simulink library "temp"  (Simulink 5.0)
undefined symbols (not defined in the file or in its folder): A, A1, B, B1, C, C1, D, D1, F, H, matrix, v1_vec, v2_vec, v3_vec, v_vec
libraries: aerolibschedule x46, simulink3 x46, simulink x18
(part 1 of 2)
settings Model: Creator=sgage  LastModifiedBy=sgage  ExtModeAutoUpdateStatusClock=off

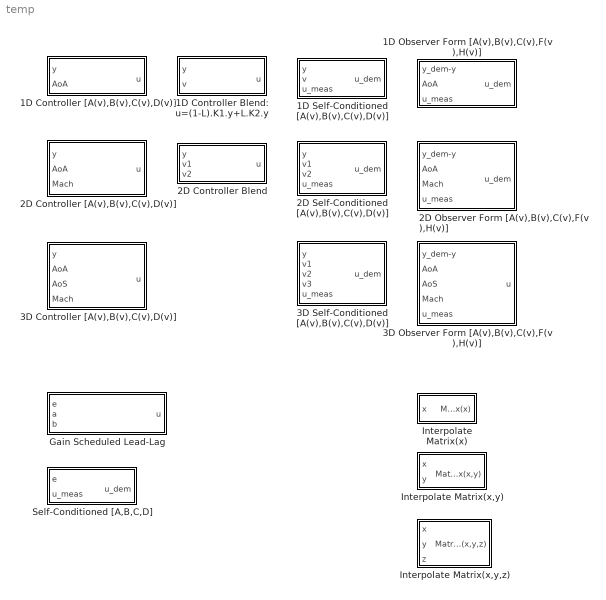
== system temp ==
  1D Controller [A(v),B(v),C(v),D(v)] : Subsystem  mask(StateSpaceABCD-1D){A=A1, B=B1, C=C1, D=D1, AoA_vec=v_vec, x_initial=0}
      mask prompts: A "A-matrix(v):"; B "B-matrix(v):"; C "C-matrix(v):"; D "D-matrix(v):"; AoA_vec "Scheduling variable breakpoints:"; x_initial "Initial state, x_initial:"
      mask help: Implement a state-space controller [A,B,C,D] where A, B, C, and D depend on one scheduling parameter, v.
      mask Help: web(asbhelp('1dcontrolleravbvcvdv'));
      mask Display:
      | port_label('input',1,'y');
      | port_label('input',2,'v');
      | port_label('output',1,'u');
  1D Controller Blend: u=(1-L).K1.y+L.K2.y : Subsystem  mask(Blend-1D){A=A1, B=B1, C=C1, D=D1, breakpoints_v=[1 1.5 2], x_initial=0, vec_w=[-5 -2]}
      mask prompts: A "A-matrix(v):"; B "B-matrix(v):"; C "C-matrix(v):"; D "D-matrix(v):"; breakpoints_v "Scheduling variable breakpoints:"; x_initial "Initial state, x_initial:"; vec_w "Poles of A(v)-H(v)*C(v) = [w1 ... wn]:"
      mask help: Blend between outputs of a 1-D vector of state-space controllers. All controllers must have the same state dimension.
      mask init:
      | for i=1:length(breakpoints_v);
      |     L1 = place(squeeze(A(:,:,i))',squeeze(C(:,:,i))',vec_w);
      |     H(:,:,i)=L1';
      | end
      mask Help: web(asbhelp('1dcontrollerblendu1l.k1.yl.k2.y'));
  1D Observer Form [A(v),B(v),C(v),F(v),H(v)] : Subsystem  mask(StateSpaceABCFH-1D){A=A, B=B, C=C, F=F, H=H, AoA_vec=v_vec, x_initial=0}
      mask prompts: A "A-matrix(v):"; B "B-matrix(v):"; C "C-matrix(v):"; F "F-matrix(v):"; H "H-matrix(v):"; AoA_vec "Scheduling variable breakpoints:"; x_initial "Initial state, x_initial:"
      mask help: Implement a state-space controller [A,B,C,F,H] in observer form where A, B, C, F, and H depend on one scheduling parameter.
      mask Help: web(asbhelp('1dobserverformavbvcvfvhv'));
      mask Display:
      | port_label('input',1,'y-y_dem');
      | port_label('input',2,'v');
      | port_label('input',3,'u_meas');
      | port_label('output',1,'u_dem')
  1D Self-Conditioned [A(v),B(v),C(v),D(v)] : Subsystem  mask(StateSpaceSelfCond-1D){A=A, B=B, C=C, D=D, breakpoints_v=v_vec, x_initial=0, vec_w=[-5 -2]}
      mask prompts: A "A-matrix(v):"; B "B-matrix(v):"; C "C-matrix(v):"; D "D-matrix(v):"; breakpoints_v "Scheduling variable breakpoints:"; x_initial "Initial state, x_initial:"; vec_w "Poles of A(v)-H(v)*C(v) = [w1 ... wn]:"
      mask help: Implement a state-space controller [A(v),B(v),C(v),D(v)] in a self-conditioned form. If u_meas = u_dem, then the implemented controller is [A,B,C,D]. If u_meas is limited, e.g., rate limiting, then the poles of the controller become those defined in the mask dialog box. Uses call to Control Systems Toolbox function place.m when initializing. A, B, C, and D should be 3-D matrices, the last dimension corresponding to the scheduling parameter, and the first two corresponding to the matrix for a given set of scheduling parameter values.
      mask init:
      | for i=1:length(breakpoints_v);
      |     L1 = place(squeeze(A(:,:,i))',squeeze(C(:,:,i))',vec_w);
      |     H(:,:,i)=L1';
      | end
      mask Help: web(asbhelp('1dselfconditionedavbvcvdv'));
  2D Controller [A(v),B(v),C(v),D(v)] : Subsystem  mask(StateSpaceABCD-2D){A=A, B=B, C=C, D=D, AoA_vec=v1_vec, Mach_vec=v2_vec, x_initial=0}
      mask prompts: A "A-matrix(v1,v2):"; B "B-matrix(v1,v2):"; C "C-matrix(v1,v2):"; D "D-matrix(v1,v2):"; AoA_vec "First scheduling variable (v1) breakpoints:"; Mach_vec "Second scheduling variable (v2) breakpoints:"; x_initial "Initial state, x_initial:"
      mask help: Implement a state-space controller [A,B,C,D] where A, B, C, and D depend on two scheduling parameters, v1 and v2.
      mask Help: web(asbhelp('2dcontrolleravbvcvdv'));
      mask Display:
      | port_label('input',1,'y');
      | port_label('input',2,'v1');
      | port_label('input',3,'v2');
      | port_label('output',1,'u');
  2D Controller Blend : Subsystem  mask(Blend-2D){A=A, B=B, C=C, D=D, breakpoints_v1=v1_vec, breakpoints_v2=v2_vec, x_initial=0, vec_w=[-5 -2]}
      mask prompts: A "A-matrix(v1,v2):"; B "B-matrix(v1,v2):"; C "C-matrix(v1,v2):"; D "D-matrix(v1,v2):"; breakpoints_v1 "First scheduling variable (v1) breakpoints:"; breakpoints_v2 "Second scheduling variable (v2) breakpoints:"; x_initial "Initial state, x_initial:"; vec_w "Poles of A(v)-H(v)*C(v) = [w1 ... wn]:"
      mask help: Blend between outputs of a 2-D vector of state-space controllers. All controllers must have the same state dimension.
      mask init:
      | for i=1:length(breakpoints_v1);
      |   for j=1:length(breakpoints_v2);
      |     L1 = place(squeeze(A(:,:,i,j))',squeeze(C(:,:,i,j))',vec_w);
      |     H(:,:,i,j)=L1';
      |   end
      | end
      mask Help: web(asbhelp('2dcontrollerblend'));
  2D Observer Form [A(v),B(v),C(v),F(v),H(v)] : Subsystem  mask(StateSpaceABCFH-2D){A=A, B=B, C=C, F=F, H=H, AoA_vec=v1_vec, Mach_vec=v2_vec, x_initial=0}
      mask prompts: A "A-matrix(v1,v2):"; B "B-matrix(v1,v2):"; C "C-matrix(v1,v2):"; F "F-matrix(v1,v2):"; H "H-matrix(v1,v2):"; AoA_vec "First scheduling variable (v1) breakpoints:"; Mach_vec "Second scheduling variable (v2) breakpoints:"; x_initial "Initial state, x_initial:"
      mask help: Implement a state-space controller [A,B,C,F,H] in observer form where A, B, C, F, and H depend on two scheduling parameters.
      mask Help: web(asbhelp('2dobserverformavbvcvfvhv'));
      mask Display:
      | port_label('input',1,'y-y_dem');
      | port_label('input',2,'v1');
      | port_label('input',3,'v2');
      | port_label('input',4,'u_meas');
      | port_label('output',1,'u_dem')
  2D Self-Conditioned [A(v),B(v),C(v),D(v)] : Subsystem  mask(StateSpaceSelfCond-2D){A=A, B=B, C=C, D=D, breakpoints_v1=v1_vec, breakpoints_v2=v2_vec, x_initial=0, vec_w=[-5 -2]}
      mask prompts: A "A-matrix(v1,v2):"; B "B-matrix(v1,v2):"; C "C-matrix(v1,v2):"; D "D-matrix(v1,v2):"; breakpoints_v1 "First scheduling variable (v1) breakpoints:"; breakpoints_v2 "Second scheduling variable (v2) breakpoints:"; x_initial "Initial state, x_initial:"; vec_w "Poles of A(v)-H(v)*C(v) = [w1 ... wn]:"
      mask help: Implement a state-space controller [A(v1,v2),B(v1,v2),C(v1,v2),D(v1,v2)] in a self-conditioned form. If u_meas = u_dem, then the implemented controller is [A,B,C,D]. If u_meas is limited, e.g., rate limiting, then the poles of the controller become those defined in the mask dialog box. Uses call to Control Systems Toolbox function place.m when initializing. A, B, C, and D should be 4-D matrices, the last two dimensions corresponding to the scheduling parameters, and the first two corresponding to the matrix for a given set of scheduling parameter values.
      mask init:
      | for i=1:length(breakpoints_v1);
      |   for j=1:length(breakpoints_v2);
      |     L1 = place(squeeze(A(:,:,i,j))',squeeze(C(:,:,i,j))',vec_w);
      |     H(:,:,i,j)=L1';
      |   end
      | end
      mask Help: web(asbhelp('2dselfconditionedavbvcvdv'));
  3D Controller [A(v),B(v),C(v),D(v)] : Subsystem  mask(StateSpaceABCD-3D){A=A, B=B, C=C, D=D, AoA_vec=v1_vec, AoS_vec=v2_vec, Mach_vec=v3_vec, x_initial=0}
      mask prompts: A "A-matrix(v1,v2,v3):"; B "B-matrix(v1,v2,v3):"; C "C-matrix(v1,v2,v3):"; D "D-matrix(v1,v2,v3):"; AoA_vec "First scheduling variable (v1) breakpoints:"; AoS_vec "Second scheduling variable (v2) breakpoints:"; Mach_vec "Third scheduling variable (v3) breakpoints:"; x_initial "Initial state, x_initial:"
      mask help: Implement a state-space controller [A,B,C,D] where A, B, C, and D depend on three scheduling parameters, v1, v2, and v3.
      mask Help: web(asbhelp('3dcontrolleravbvcvdv'));
      mask Display:
      | port_label('input',1,'y');
      | port_label('input',2,'v1');
      | port_label('input',3,'v2');
      | port_label('input',4,'v3');
      | port_label('output',1,'u');
  3D Observer Form [A(v),B(v),C(v),F(v),H(v)] : Subsystem  mask(StateSpaceABCFH-3D){A=A, B=B, C=C, F=F, H=H, AoA_vec=v1_vec, AoS_vec=v2_vec, Mach_vec=v3_vec, x_initial=0}
      mask prompts: A "A-matrix(v1,v2,v3):"; B "B-matrix(v1,v2,v3):"; C "C-matrix(v1,v2,v3):"; F "F-matrix(v1,v2,v3):"; H "H-matrix(v1,v2,v3):"; AoA_vec "First scheduling variable (v1) breakpoints:"; AoS_vec "Second scheduling variable (v2) breakpoints:"; Mach_vec "Third scheduling variable (v3) breakpoints:"; x_initial "Initial state, x_initial:"
      mask help: Implement a state-space controller [A,B,C,F,H] in observer form where A, B, C, F, and H depend on three scheduling parameters.
      mask Help: web(asbhelp('3dobserverformavbvcvfvhv'));
      mask Display:
      | port_label('input',1,'y-y_dem');
      | port_label('input',2,'v1');
      | port_label('input',3,'v2');
      | port_label('input',4,'v3');
      | port_label('input',5,'u_meas');
      | port_label('output',1,'u_dem')
  3D Self-Conditioned [A(v),B(v),C(v),D(v)] : Subsystem  mask(StateSpaceSelfCond-3D){A=A, B=B, C=C, D=D, breakpoints_v1=v1_vec, breakpoints_v2=v2_vec, breakpoints_v3=v3_vec, x_initial=0, vec_w=[-5 -2]}
      mask prompts: A "A-matrix(v1,v2,v3):"; B "B-matrix(v1,v2,v3):"; C "C-matrix(v1,v2,v3):"; D "D-matrix(v1,v2,v3):"; breakpoints_v1 "First scheduling variable (v1) breakpoints:"; breakpoints_v2 "Second scheduling variable (v2) breakpoints:"; breakpoints_v3 "Third scheduling variable (v3) breakpoints:"; x_initial "Initial state, x_initial:"; vec_w "Poles of A(v)-H(v)*C(v) = [w1 ... wn]:"
      mask help: Implement a state-space controller [A(v1,v2,v3),B(v1,v2,v3),C(v1,v2,v3),D(v1,v2,v3)] in a self-conditioned form. If u_meas = u_dem, then the implemented controller is [A,B,C,D]. If u_meas is limited, e.g., rate limiting, then the poles of the controller become those defined in the mask dialog box. Uses call to Control Systems Toolbox function place.m when initializing. A, B, C, and D should be 5-D matrices, the last three dimensions corresponding to the scheduling parameters, and the first two corresponding to the matrix for a given set of scheduling parameter values.
      mask init:
      | for i=1:length(breakpoints_v1);
      |   for j=1:length(breakpoints_v2);
      |     for k=1:length(breakpoints_v3);
      |       L1 = place(squeeze(A(:,:,i,j,k))',squeeze(C(:,:,i,j,k))',vec_w);
      |       H(:,:,i,j,k)=L1';
      |     end
      |   end
      | end
      mask Help: web(asbhelp('3dselfconditionedavbvcvdv'));
  Gain Scheduled Lead-Lag : Subsystem  mask(Gain Scheduled Lead-Lag){x_initial=0}
      mask prompts: x_initial "Initial state, x_initial:"
      mask help: Implement gain-scheduled first-order lead-lag of the form [1+a.s]/[1+b.s]. Initial output is given by (x_initial+a.e)/b where x_initial is the initial state defined in the mask dialog box. Note that b should never be allowed to be zero.
      mask Help: web(asbhelp);
      mask Display:
      | port_label('input',1,'e');
      | port_label('input',2,'a');
      | port_label('input',3,'b');
      | port_label('output',1,'u');
      | disp('(1+a.s)/(1+b.s)')
  Interpolate Matrix(x) : Subsystem  mask(MatrixSchedule-1D){matrix=matrix}
      mask prompts: matrix "Matrix to interpolate:"
      mask help: Return an interpolated matrix for given input x. Input x must be from the Simulink PreLook-up Index Search block.
      mask Help: web(asbhelp('interpolatematrixx'));
  Interpolate Matrix(x,y) : Subsystem  mask(MatrixSchedule-2D){matrix=matrix}
      mask prompts: matrix "Matrix to interpolate:"
      mask help: Return an interpolated matrix for given inputs x and y. Inputs x and y must be from Simulink PreLook-up Index Search block.
      mask Help: web(asbhelp('interpolatematrixxy'));
  Interpolate Matrix(x,y,z) : Subsystem  mask(MatrixSchedule-3D){matrix=matrix}
      mask prompts: matrix "Matrix to interpolate:"
      mask help: Return an interpolated matrix for given inputs x, y, and z. Inputs x, y, z must be from Simulink PreLook-up Index Search block.
      mask Help: web(asbhelp('interpolatematrixxyz'));
  Self-Conditioned [A,B,C,D] : Subsystem  mask(Self-Conditioned){Ak=[-1 -0.2;0 -3], Bk=[1;1], Ck=[1 0], Dk=0.02, x_initial=0, vec_w=[-5 -2]}
      mask prompts: Ak "A-matrix:"; Bk "B-matrix:"; Ck "C-matrix:"; Dk "D-matrix:"; x_initial "Initial state, x_initial:"; vec_w "Poles of A-H*C = [w1 ... wn]:"
      mask help: Implement a state-space controller [A,B,C,D] in a self-conditioned form. If u_meas = u_dem, then the implemented controller is [A,B,C,D]. If u_meas is limited, e.g., rate limiting, then the poles of the controller become those defined in the mask dialog box. Uses call to Control Systems Toolbox function place.m when initializing.
      mask init:
      | L1 = place(Ak',Ck',vec_w);
      | H=L1';
      mask Help: web(asbhelp('selfconditionedabcd'))

== system temp/1D Controller [A(v),B(v),C(v),D(v)] ==
  y : Inport
  AoA : Inport  Port=2  PortDimensions=1
  "[A,B,C,D]" : Subsystem
  alpha (degs) : simulink3/Functions & Tables/PreLook-Up Index Search  bpData=AoA_vec  searchMode=Binary Search  cacheBpFlag=on  outputFlag=off  extrapMode=Clip to Range  rangeErrorMode=None
  u : Outport
  wires:
  y/1 -> "[A,B,C,D]"/1(y)
  AoA/1 -> alpha (degs)/1
  alpha (degs)/1 -> "[A,B,C,D]"/2(AoA)
  "[A,B,C,D]"/1(u) -> u/1

== system temp/1D Controller Blend: u=(1-L).K1.y+L.K2.y ==
  y : Inport
  v : Inport  Port=2  PortDimensions=1
  Breakpoints : simulink/Look-Up Tables/PreLook-Up Index Search  bpData=breakpoints_v  searchMode=Binary Search  cacheBpFlag=on  outputFlag=off  extrapMode=Clip to Range  rangeErrorMode=None
  Controller indices : Subsystem  AncestorBlock=|
      | aerolibschedule/1D Controller Blend:
      | u=(1-L).K1.y+L.K2.y/Controller indices
  Demux : Demux  Outputs=2
  K1 : Subsystem
  K2 : Subsystem
  K3 : Subsystem
  Sum1 : Sum  Inputs=+++  SaturateOnIntegerOverflow=on  InputSameDT=on
  lambda1 : Product  SaturateOnIntegerOverflow=on  InputSameDT=on
  lambda2 : Product  SaturateOnIntegerOverflow=on  InputSameDT=on
  lambda3 : Product  SaturateOnIntegerOverflow=on  InputSameDT=on
  u : Outport
  wires:
  Controller indices/6(lambda_K3) -> lambda3/2
  Controller indices/4(lambda_K2) -> lambda2/2
  Controller indices/2(lambda_K1) -> lambda1/2
  Sum1/1 -> K1/3(u_measured), K3/3(u_measured), K2/3(u_measured), u/1
  lambda3/1 -> Sum1/3
  lambda1/1 -> Sum1/1
  lambda2/1 -> Sum1/2
  K3/1(u_demand) -> lambda3/1
  K2/1(u_demand) -> lambda2/1
  K1/1(u_demand) -> lambda1/1
  Controller indices/5(idx_K3) -> K3/2(index)
  Controller indices/3(idx_K2) -> K2/2(index)
  Controller indices/1(idx_K1) -> K1/2(index)
  Demux/2 -> Controller indices/2(lambda)
  Demux/1 -> Controller indices/1(index)
  Breakpoints/1 -> Demux/1
  v/1 -> Breakpoints/1
  y/1 -> K1/1(e = refs - y), K3/1(e = refs - y), K2/1(e = refs - y)

== system temp/1D Observer Form [A(v),B(v),C(v),F(v),H(v)] ==
  y_dem-y : Inport
  AoA : Inport  Port=2  PortDimensions=1
  u_meas : Inport  Port=3
  Reshape : simulink3/Signals & Systems/Reshape  OutputDimensionality=1-D array  OutputDimensions=[1,1]
  Reshape1 : simulink3/Signals & Systems/Reshape  OutputDimensionality=Column vector  OutputDimensions=[1,1]
  Reshape2 : simulink3/Signals & Systems/Reshape  OutputDimensionality=Column vector  OutputDimensions=[1,1]
  "[A,B,C,F,H]" : Subsystem
  alpha (degs) : simulink3/Functions & Tables/PreLook-Up Index Search  bpData=AoA_vec  searchMode=Binary Search  cacheBpFlag=on  outputFlag=off  extrapMode=Clip to Range  rangeErrorMode=None
  u_dem : Outport
  wires:
  "[A,B,C,F,H]"/1(u_dem) -> Reshape/1
  AoA/1 -> alpha (degs)/1
  y_dem-y/1 -> Reshape2/1
  alpha (degs)/1 -> "[A,B,C,F,H]"/2(AoA)
  u_meas/1 -> Reshape1/1
  Reshape/1 -> u_dem/1
  Reshape1/1 -> "[A,B,C,F,H]"/3(u_meas)
  Reshape2/1 -> "[A,B,C,F,H]"/1(y-y_dem)

== system temp/1D Self-Conditioned [A(v),B(v),C(v),D(v)] ==
  y : Inport
  v : Inport  Port=2  PortDimensions=1
  u_meas : Inport  Port=3
  Breakpoints : simulink3/Functions & Tables/PreLook-Up Index Search  bpData=breakpoints_v  searchMode=Binary Search  cacheBpFlag=on  outputFlag=off  extrapMode=Clip to Range  rangeErrorMode=None
  Controller : Subsystem
  u_dem : Outport
  wires:
  v/1 -> Breakpoints/1
  y/1 -> Controller/1(y)
  Controller/1(u_demand) -> u_dem/1
  Breakpoints/1 -> Controller/2(idx_v,lam_v)
  u_meas/1 -> Controller/3(u_measured)

== system temp/2D Controller [A(v),B(v),C(v),D(v)] ==
  y : Inport
  AoA : Inport  Port=2  PortDimensions=1
  Mach : Inport  Port=3  PortDimensions=1
  Mach No. : simulink3/Functions & Tables/PreLook-Up Index Search  bpData=Mach_vec  searchMode=Binary Search  cacheBpFlag=on  outputFlag=off  extrapMode=Clip to Range  rangeErrorMode=None
  "[A,B,C,D]" : Subsystem
  alpha (degs) : simulink3/Functions & Tables/PreLook-Up Index Search  bpData=AoA_vec  searchMode=Binary Search  cacheBpFlag=on  outputFlag=off  extrapMode=Clip to Range  rangeErrorMode=None
  u : Outport
  wires:
  y/1 -> "[A,B,C,D]"/1(y)
  Mach/1 -> Mach No./1
  AoA/1 -> alpha (degs)/1
  Mach No./1 -> "[A,B,C,D]"/3(Mach)
  alpha (degs)/1 -> "[A,B,C,D]"/2(AoA)
  "[A,B,C,D]"/1(u) -> u/1

== system temp/2D Controller Blend ==
  y : Inport
  v1 : Inport  Port=2  PortDimensions=1
  v2 : Inport  Port=3  PortDimensions=1
  Breakpoints v1 : simulink/Look-Up Tables/PreLook-Up Index Search  bpData=breakpoints_v1  searchMode=Binary Search  cacheBpFlag=on  outputFlag=off  extrapMode=Clip to Range  rangeErrorMode=None
  Controller indices1 : Subsystem
  Demux : Demux  Outputs=2
  K1 : Subsystem
  K2 : aerolibschedule/2D Controller Blend/K1  SimViewingDevice=off  DataTypeOverride=UseLocalSettings  MinMaxOverflowLogging=UseLocalSettings
      settings: Permissions=ReadWrite  RTWFcnNameOpts=Auto  RTWFileNameOpts=Auto
  K3 : aerolibschedule/2D Controller Blend/K1  SimViewingDevice=off  DataTypeOverride=UseLocalSettings  MinMaxOverflowLogging=UseLocalSettings
      settings: Permissions=ReadWrite  RTWFcnNameOpts=Auto  RTWFileNameOpts=Auto
  Sum1 : Sum  Inputs=+++  SaturateOnIntegerOverflow=on  InputSameDT=on
  lambda1 : Product  SaturateOnIntegerOverflow=on  InputSameDT=on
  lambda2 : Product  SaturateOnIntegerOverflow=on  InputSameDT=on
  lambda3 : Product  SaturateOnIntegerOverflow=on  InputSameDT=on
  u : Outport
  wires:
  v2/1 -> K2/4, K3/4, K1/4(v2)
  Controller indices1/6(lambda_K3) -> lambda3/2
  Controller indices1/4(lambda_K2) -> lambda2/2
  Controller indices1/2(lambda_K1) -> lambda1/2
  Sum1/1 -> K2/3, K3/3, K1/3(u_measured), u/1
  lambda3/1 -> Sum1/3
  lambda1/1 -> Sum1/1
  lambda2/1 -> Sum1/2
  K3/1 -> lambda3/1
  K2/1 -> lambda2/1
  K1/1(u_demand) -> lambda1/1
  Controller indices1/5(idx_K3) -> K3/2
  Controller indices1/3(idx_K2) -> K2/2
  Controller indices1/1(idx_K1) -> K1/2(index_v1)
  Demux/2 -> Controller indices1/2(lambda)
  Demux/1 -> Controller indices1/1(index)
  Breakpoints v1/1 -> Demux/1
  v1/1 -> Breakpoints v1/1
  y/1 -> K2/1, K3/1, K1/1(e = refs - y)

== system temp/2D Observer Form [A(v),B(v),C(v),F(v),H(v)] ==
  y_dem-y : Inport
  AoA : Inport  Port=2  PortDimensions=1
  Mach : Inport  Port=3  PortDimensions=1
  u_meas : Inport  Port=4
  Mach No. : simulink3/Functions & Tables/PreLook-Up Index Search  bpData=Mach_vec  searchMode=Binary Search  cacheBpFlag=on  outputFlag=off  extrapMode=Clip to Range  rangeErrorMode=None
  Reshape : simulink3/Signals & Systems/Reshape  OutputDimensionality=1-D array  OutputDimensions=[1,1]
  Reshape1 : simulink3/Signals & Systems/Reshape  OutputDimensionality=Column vector  OutputDimensions=[1,1]
  Reshape2 : simulink3/Signals & Systems/Reshape  OutputDimensionality=Column vector  OutputDimensions=[1,1]
  "[A,B,C,F,H]" : Subsystem
  alpha (degs) : simulink3/Functions & Tables/PreLook-Up Index Search  bpData=AoA_vec  searchMode=Binary Search  cacheBpFlag=on  outputFlag=off  extrapMode=Clip to Range  rangeErrorMode=None
  u_dem : Outport
  wires:
  "[A,B,C,F,H]"/1(u_dem) -> Reshape/1
  alpha (degs)/1 -> "[A,B,C,F,H]"/2(AoA)
  Mach No./1 -> "[A,B,C,F,H]"/3(Mach)
  AoA/1 -> alpha (degs)/1
  Mach/1 -> Mach No./1
  y_dem-y/1 -> Reshape1/1
  u_meas/1 -> Reshape2/1
  Reshape/1 -> u_dem/1
  Reshape1/1 -> "[A,B,C,F,H]"/1(y-y_dem)
  Reshape2/1 -> "[A,B,C,F,H]"/4(u_meas)

== system temp/2D Self-Conditioned [A(v),B(v),C(v),D(v)] ==
  y : Inport
  v1 : Inport  Port=2  PortDimensions=1
  v2 : Inport  Port=3  PortDimensions=1
  u_meas : Inport  Port=4
  Breakpoints v1 : simulink3/Functions & Tables/PreLook-Up Index Search  bpData=breakpoints_v1  searchMode=Binary Search  cacheBpFlag=on  outputFlag=off  extrapMode=Clip to Range  rangeErrorMode=None
  Breakpoints v2 : simulink3/Functions & Tables/PreLook-Up Index Search  bpData=breakpoints_v2  searchMode=Binary Search  cacheBpFlag=on  outputFlag=off  extrapMode=Clip to Range  rangeErrorMode=None
  Controller : Subsystem
  u_dem : Outport
  wires:
  u_meas/1 -> Controller/4(u_measured)
  Breakpoints v1/1 -> Controller/2(idx_v1,lam_v1)
  Controller/1(u_demand) -> u_dem/1
  y/1 -> Controller/1(y)
  v1/1 -> Breakpoints v1/1
  v2/1 -> Breakpoints v2/1
  Breakpoints v2/1 -> Controller/3(idx_v2,lam_v2)

== system temp/3D Controller [A(v),B(v),C(v),D(v)] ==
  y : Inport
  AoA : Inport  Port=2  PortDimensions=1
  AoS : Inport  Port=3  PortDimensions=1
  Mach : Inport  Port=4  PortDimensions=1
  Mach No. : simulink3/Functions & Tables/PreLook-Up Index Search  bpData=Mach_vec  searchMode=Binary Search  cacheBpFlag=on  outputFlag=off  extrapMode=Clip to Range  rangeErrorMode=None
  "[A,B,C,D]" : Subsystem
  alpha (degs) : simulink3/Functions & Tables/PreLook-Up Index Search  bpData=AoA_vec  searchMode=Binary Search  cacheBpFlag=on  outputFlag=off  extrapMode=Clip to Range  rangeErrorMode=None
  beta (degs) : simulink3/Functions & Tables/PreLook-Up Index Search  bpData=AoS_vec  searchMode=Binary Search  cacheBpFlag=on  outputFlag=off  extrapMode=Clip to Range  rangeErrorMode=None
  u : Outport
  wires:
  "[A,B,C,D]"/1(u) -> u/1
  alpha (degs)/1 -> "[A,B,C,D]"/2(AoA)
  beta (degs)/1 -> "[A,B,C,D]"/3(AoS)
  Mach No./1 -> "[A,B,C,D]"/4(Mach)
  AoA/1 -> alpha (degs)/1
  AoS/1 -> beta (degs)/1
  Mach/1 -> Mach No./1
  y/1 -> "[A,B,C,D]"/1(y)

== system temp/3D Observer Form [A(v),B(v),C(v),F(v),H(v)] ==
  y_dem-y : Inport
  AoA : Inport  Port=2  PortDimensions=1
  AoS : Inport  Port=3  PortDimensions=1
  Mach : Inport  Port=4  PortDimensions=1
  u_meas : Inport  Port=5
  Mach No. : simulink3/Functions & Tables/PreLook-Up Index Search  bpData=Mach_vec  searchMode=Binary Search  cacheBpFlag=on  outputFlag=off  extrapMode=Clip to Range  rangeErrorMode=None
  Reshape : simulink3/Signals & Systems/Reshape  OutputDimensionality=1-D array  OutputDimensions=[1,1]
  Reshape1 : simulink3/Signals & Systems/Reshape  OutputDimensionality=Column vector  OutputDimensions=[1,1]
  Reshape2 : simulink3/Signals & Systems/Reshape  OutputDimensionality=Column vector  OutputDimensions=[1,1]
  "[A,B,C,F,H]" : Subsystem
  alpha (degs) : simulink3/Functions & Tables/PreLook-Up Index Search  bpData=AoA_vec  searchMode=Binary Search  cacheBpFlag=on  outputFlag=off  extrapMode=Clip to Range  rangeErrorMode=None
  beta (degs) : simulink3/Functions & Tables/PreLook-Up Index Search  bpData=AoS_vec  searchMode=Binary Search  cacheBpFlag=on  outputFlag=off  extrapMode=Clip to Range  rangeErrorMode=None
  u : Outport
  wires:
  y_dem-y/1 -> Reshape1/1
  Mach/1 -> Mach No./1
  AoS/1 -> beta (degs)/1
  AoA/1 -> alpha (degs)/1
  Mach No./1 -> "[A,B,C,F,H]"/4(Mach)
  beta (degs)/1 -> "[A,B,C,F,H]"/3(AoS)
  alpha (degs)/1 -> "[A,B,C,F,H]"/2(AoA)
  "[A,B,C,F,H]"/1(u_dem) -> Reshape/1
  u_meas/1 -> Reshape2/1
  Reshape/1 -> u/1
  Reshape1/1 -> "[A,B,C,F,H]"/1(y-y_dem)
  Reshape2/1 -> "[A,B,C,F,H]"/5(u_meas)

== system temp/3D Self-Conditioned [A(v),B(v),C(v),D(v)] ==
  y : Inport
  v1 : Inport  Port=2  PortDimensions=1
  v2 : Inport  Port=3  PortDimensions=1
  v3 : Inport  Port=4  PortDimensions=1
  u_meas : Inport  Port=5
  Breakpoints v1 : simulink3/Functions & Tables/PreLook-Up Index Search  bpData=breakpoints_v1  searchMode=Binary Search  cacheBpFlag=on  outputFlag=off  extrapMode=Clip to Range  rangeErrorMode=None
  Breakpoints v2 : simulink3/Functions & Tables/PreLook-Up Index Search  bpData=breakpoints_v2  searchMode=Binary Search  cacheBpFlag=on  outputFlag=off  extrapMode=Clip to Range  rangeErrorMode=None
  Breakpoints v3 : simulink3/Functions & Tables/PreLook-Up Index Search  bpData=breakpoints_v3  searchMode=Binary Search  cacheBpFlag=on  outputFlag=off  extrapMode=Clip to Range  rangeErrorMode=None
  Controller : Subsystem
  u_dem : Outport
  wires:
  Breakpoints v2/1 -> Controller/3(idx_v2,lam_v2)
  v2/1 -> Breakpoints v2/1
  v1/1 -> Breakpoints v1/1
  y/1 -> Controller/1(y)
  Controller/1(u_demand) -> u_dem/1
  Breakpoints v1/1 -> Controller/2(idx_v1,lam_v1)
  u_meas/1 -> Controller/5(u_measured)
  v3/1 -> Breakpoints v3/1
  Breakpoints v3/1 -> Controller/4(idx_v3,lam_v3)

== system temp/Gain Scheduled Lead-Lag ==
  e : Inport  PortDimensions=1
  a : Inport  Port=2  PortDimensions=1
  b : Inport  Port=3  PortDimensions=1
  Integrator : Integrator  InitialCondition=x_initial
  Product : Product  SaturateOnIntegerOverflow=on  InputSameDT=on
  Product1 : Product  Inputs=*/  SaturateOnIntegerOverflow=on  InputSameDT=on
  Sum : Sum  Inputs=|+-  SaturateOnIntegerOverflow=on  InputSameDT=on
  Sum1 : Sum  Inputs=++|  SaturateOnIntegerOverflow=on  InputSameDT=on
  u : Outport
  wires:
  Sum/1 -> Integrator/1
  e/1 -> Sum/1, Product/2
  Integrator/1 -> Sum1/2
  Product/1 -> Sum1/1
  a/1 -> Product/1
  Sum1/1 -> Product1/1
  b/1 -> Product1/2
  Product1/1 -> u/1, Sum/2

== system temp/Interpolate Matrix(x) ==
  x : Inport
  Demux : Demux  Outputs=[1,1]
  Matrix interpolation : Subsystem
  Matrix(x) : Outport
  wires:
  Matrix interpolation/1(matrix) -> Matrix(x)/1
  Demux/2 -> Matrix interpolation/2(lambda_x)
  Demux/1 -> Matrix interpolation/1(index)
  x/1 -> Demux/1

== system temp/Interpolate Matrix(x,y) ==
  x : Inport
  y : Inport  Port=2
  Demux : Demux  Outputs=2
  Demux1 : Demux  Outputs=2
  Matrix interpolation : Subsystem
  Mux2 : Mux  Inputs=2
  Matrix(x,y) : Outport
  wires:
  x/1 -> Demux/1
  y/1 -> Demux1/1
  Demux/1 -> Mux2/1
  Demux1/1 -> Mux2/2
  Mux2/1 -> Matrix interpolation/1(indices)
  Demux/2 -> Matrix interpolation/2(lambda_x)
  Demux1/2 -> Matrix interpolation/3(lambda_y)
  Matrix interpolation/1(matrix) -> Matrix(x,y)/1

== system temp/Interpolate Matrix(x,y,z) ==
  x : Inport
  y : Inport  Port=2
  z : Inport  Port=3
  1-lambda_z : Product  SaturateOnIntegerOverflow=on  InputSameDT=on
  Demux : Demux  Outputs=2
  Demux1 : Demux  Outputs=2
  Demux2 : Demux  Outputs=2
  Fcn1 : Fcn  Expr=1-u(1)
  Matrix for lambda_z=0 : Subsystem
  Matrix for lambda_z=1 : Subsystem
  Mux2 : Mux  Inputs=3
  Sum5 : Sum  Inputs=+|+  SaturateOnIntegerOverflow=on  InputSameDT=on
  lambda_z : Product  SaturateOnIntegerOverflow=on  InputSameDT=on
  Matrix(x,y,z) : Outport
  wires:
  Sum5/1 -> Matrix(x,y,z)/1
  Matrix for lambda_z=0/1(matrix) -> 1-lambda_z/1
  Matrix for lambda_z=1/1(matrix) -> lambda_z/1
  Fcn1/1 -> 1-lambda_z/2
  1-lambda_z/1 -> Sum5/1
  lambda_z/1 -> Sum5/2
  Demux1/2 -> Matrix for lambda_z=0/3(lambda_y), Matrix for lambda_z=1/3(lambda_y)
  Demux/2 -> Matrix for lambda_z=0/2(lambda_x), Matrix for lambda_z=1/2(lambda_x)
  Mux2/1 -> Matrix for lambda_z=0/1(indices), Matrix for lambda_z=1/1(indices)
  Demux2/1 -> Mux2/3
  Demux1/1 -> Mux2/2
  Demux/1 -> Mux2/1
  z/1 -> Demux2/1
  y/1 -> Demux1/1
  x/1 -> Demux/1
  Demux2/2 -> lambda_z/2, Fcn1/1

== system temp/Self-Conditioned [A,B,C,D] ==
  e : Inport
  u_meas : Inport  Port=2
  Ak-H*Ck : Gain  Orientation=left  Gain=Ak-H*Ck  Multiplication=Matrix(K*u)  SaturateOnIntegerOverflow=on
  Bk-H*Dk : Gain  Gain=Bk-H*Dk  Multiplication=Matrix(K*u)  SaturateOnIntegerOverflow=on
  Ck : Gain  Gain=Ck  Multiplication=Matrix(K*u)  SaturateOnIntegerOverflow=on
  Dk : Gain  Gain=Dk  Multiplication=Matrix(K*u)  SaturateOnIntegerOverflow=on
  H : Gain  Gain=H  Multiplication=Matrix(K*u)  SaturateOnIntegerOverflow=on
  Integrator : Integrator  InitialCondition=x_initial
  Sum : Sum  Inputs=|++  SaturateOnIntegerOverflow=on  InputSameDT=on
  Sum1 : Sum  Inputs=++|  SaturateOnIntegerOverflow=on  InputSameDT=on
  Sum2 : Sum  Orientation=up  Inputs=|++  SaturateOnIntegerOverflow=on  InputSameDT=on
  u_dem : Outport
  wires:
  Sum1/1 -> u_dem/1
  u_meas/1 -> H/1
  H/1 -> Sum2/1
  Ak-H*Ck/1 -> Sum2/2
  Sum2/1 -> Sum/2
  Dk/1 -> Sum1/1
  e/1 -> Dk/1, Bk-H*Dk/1
  Ck/1 -> Sum1/2
  Integrator/1 -> Ck/1, Ak-H*Ck/1
  Sum/1 -> Integrator/1
  Bk-H*Dk/1 -> Sum/1

== system temp/1D Controller [A(v),B(v),C(v),D(v)]/[A,B,C,D] ==
  y : Inport  Orientation=left
  AoA : Inport  Port=2  PortDimensions=2
  *A : Product  Multiplication=Matrix(*)  SaturateOnIntegerOverflow=on  InputSameDT=on
  *B : Product  Orientation=left  Multiplication=Matrix(*)  SaturateOnIntegerOverflow=on  InputSameDT=on
  *C : Product  Orientation=left  Multiplication=Matrix(*)  SaturateOnIntegerOverflow=on  InputSameDT=on
  *D : Product  Orientation=left  Multiplication=Matrix(*)  SaturateOnIntegerOverflow=on  InputSameDT=on
  A : aerolibschedule/Interpolate Matrix(x)  matrix=A
  B : aerolibschedule/Interpolate Matrix(x)  matrix=B
  C : aerolibschedule/Interpolate Matrix(x)  matrix=C
  D : aerolibschedule/Interpolate Matrix(x)  matrix=D
  Estimated state : Integrator  Orientation=left  InitialCondition=x_initial
  Sum : Sum  Orientation=left  Inputs=|++  SaturateOnIntegerOverflow=on  InputSameDT=on
  Sum2 : Sum  Orientation=left  Inputs=|++  SaturateOnIntegerOverflow=on  InputSameDT=on
  u : Outport  Orientation=left
  wires:
  D/1 -> *D/1
  Sum2/1 -> u/1
  *D/1 -> Sum2/2
  *C/1 -> Sum2/1
  AoA/1 -> C/1, A/1, D/1, B/1
  y/1 -> *D/2, *B/2
  B/1 -> *B/1
  C/1 -> *C/1
  A/1 -> *A/1
  *B/1 -> Sum/1
  *A/1 -> Sum/2
  Estimated state/1 -> *A/2, *C/2
  Sum/1 -> Estimated state/1

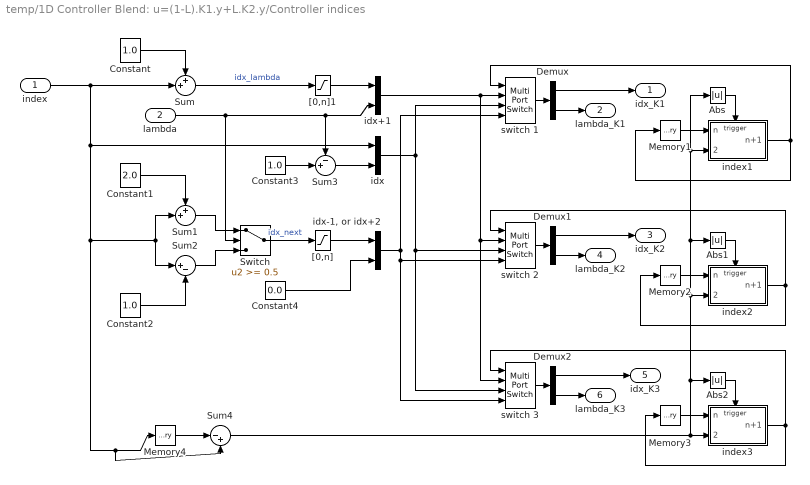
== system temp/1D Controller Blend: u=(1-L).K1.y+L.K2.y/Controller indices ==
  index : Inport
  lambda : Inport  Port=2
  Abs : Abs  SaturateOnIntegerOverflow=on
  Abs1 : Abs  SaturateOnIntegerOverflow=on
  Abs2 : Abs  SaturateOnIntegerOverflow=on
  Constant : Constant  Value=1.0
  Constant1 : Constant  Value=2.0
  Constant2 : Constant  Value=1.0
  Constant3 : Constant  Value=1.0
  Constant4 : Constant  Value=0.0
  Demux : Demux  Outputs=2
  Demux1 : Demux  Outputs=2
  Demux2 : Demux  Outputs=2
  Memory{1..4} (4 alike) : Memory
  Sum : Sum  Inputs=++|  SaturateOnIntegerOverflow=on  InputSameDT=on
  Sum1 : Sum  Inputs=++|  SaturateOnIntegerOverflow=on  InputSameDT=on
  Sum2 : Sum  Inputs=|+-  SaturateOnIntegerOverflow=on  InputSameDT=on
  Sum3 : Sum  Inputs=-+|  SaturateOnIntegerOverflow=on  InputSameDT=on
  Sum4 : Sum  Inputs=|-+  SaturateOnIntegerOverflow=on  InputSameDT=on
  Switch : Switch  Threshold=0.5  SaturateOnIntegerOverflow=on  InputSameDT=on
  "[0,n]" : Saturate  UpperLimit=length(breakpoints_v)-1  LowerLimit=0
  "[0,n]1" : Saturate  UpperLimit=length(breakpoints_v)-1  LowerLimit=0
  idx : Mux  Inputs=2
  idx+1 : Mux  Inputs=2
  "idx-1, or idx+2" : Mux  Inputs=2
  index1 : Subsystem  TreatAsAtomicUnit=on
  index2 : Subsystem  TreatAsAtomicUnit=on
  index3 : Subsystem  TreatAsAtomicUnit=on
  switch 1 : MultiPortSwitch  Inputs=3  ShowAdditionalParam=on  SaturateOnIntegerOverflow=on  InputSameDT=on
  switch 2 : MultiPortSwitch  Inputs=3  ShowAdditionalParam=on  SaturateOnIntegerOverflow=on  InputSameDT=on
  switch 3 : MultiPortSwitch  Inputs=3  ShowAdditionalParam=on  SaturateOnIntegerOverflow=on  InputSameDT=on
  idx_K1 : Outport
  lambda_K1 : Outport  Port=2
  idx_K2 : Outport  Port=3
  lambda_K2 : Outport  Port=4
  idx_K3 : Outport  Port=5
  lambda_K3 : Outport  Port=6
  wires:
  Abs2/1 -> index3/Trigger
  Abs1/1 -> index2/Trigger
  Abs/1 -> index1/Trigger
  Sum4/1 -> Abs2/1, Abs1/1, Abs/1, index1/2(rise/fall), index2/2(rise/fall), index3/2(rise/fall)
  Memory4/1 -> Sum4/1
  "[0,n]1"/1 -> idx+1/1
  "[0,n]"/1 -> "idx-1, or idx+2"/1
  Demux2/2 -> lambda_K3/1
  Demux2/1 -> idx_K3/1
  switch 3/1 -> Demux2/1
  Demux1/2 -> lambda_K2/1
  Demux1/1 -> idx_K2/1
  switch 2/1 -> Demux1/1
  Demux/2 -> lambda_K1/1
  Demux/1 -> idx_K1/1
  switch 1/1 -> Demux/1
  "idx-1, or idx+2"/1 -> switch 3/4, switch 2/4, switch 1/4
  Constant4/1 -> "idx-1, or idx+2"/2
  Switch/1 -> "[0,n]"/1  "idx_next"
  idx/1 -> switch 3/3, switch 2/3, switch 1/3
  Constant3/1 -> Sum3/2
  Sum3/1 -> idx/2
  idx+1/1 -> switch 3/2, switch 2/2, switch 1/2
  lambda/1 -> Switch/2, Sum3/1, idx+1/2
  Sum/1 -> "[0,n]1"/1  "idx_lambda"
  index3/1(n+1) -> Memory3/1, switch 3/1
  index2/1(n+1) -> Memory2/1, switch 2/1
  Memory3/1 -> index3/1(n)
  Memory2/1 -> index2/1(n)
  index1/1(n+1) -> Memory1/1, switch 1/1
  Memory1/1 -> index1/1(n)
  Constant2/1 -> Sum2/2
  Sum2/1 -> Switch/3
  Sum1/1 -> Switch/1
  Constant1/1 -> Sum1/1
  Constant/1 -> Sum/1
  index/1 -> Sum4/2, Memory4/1, Sum2/1, Sum1/2, idx/1, Sum/2

== system temp/1D Controller Blend: u=(1-L).K1.y+L.K2.y/K1 ==
  e = refs - y : Inport  Orientation=left
  index : Inport  Port=2
  u_measured : Inport  Orientation=left  Port=3
  *A-HC : Product  Multiplication=Matrix(*)  SaturateOnIntegerOverflow=on  InputSameDT=on
  *B-HD : Product  Orientation=left  Multiplication=Matrix(*)  SaturateOnIntegerOverflow=on  InputSameDT=on
  *C : Product  Orientation=left  Multiplication=Matrix(*)  SaturateOnIntegerOverflow=on  InputSameDT=on
  *D : Product  Orientation=left  Multiplication=Matrix(*)  SaturateOnIntegerOverflow=on  InputSameDT=on
  *H : Product  Orientation=left  Multiplication=Matrix(*)  SaturateOnIntegerOverflow=on  InputSameDT=on
  A : simulink/Look-Up Tables/Direct Look-Up Table (n-D)  maskTabDims=3  explicitNumDims=3  outDims=2-D Matrix  tabIsInput=off  mxTable=A  clipFlag=Warning
  B : simulink/Look-Up Tables/Direct Look-Up Table (n-D)  maskTabDims=3  explicitNumDims=3  outDims=2-D Matrix  tabIsInput=off  mxTable=B  clipFlag=Warning
  C : simulink/Look-Up Tables/Direct Look-Up Table (n-D)  maskTabDims=3  explicitNumDims=3  outDims=2-D Matrix  tabIsInput=off  mxTable=C  clipFlag=Warning
  D : simulink/Look-Up Tables/Direct Look-Up Table (n-D)  maskTabDims=3  explicitNumDims=3  outDims=2-D Matrix  tabIsInput=off  mxTable=D  clipFlag=Warning
  Estimated state : Integrator  Orientation=left  InitialCondition=x_initial
  H : simulink/Look-Up Tables/Direct Look-Up Table (n-D)  maskTabDims=3  explicitNumDims=3  outDims=2-D Matrix  tabIsInput=off  mxTable=H  clipFlag=Warning
  H*C : Product  Multiplication=Matrix(*)  SaturateOnIntegerOverflow=on  InputSameDT=on
  H*D : Product  Multiplication=Matrix(*)  SaturateOnIntegerOverflow=on  InputSameDT=on
  Sum : Sum  Orientation=left  Inputs=+++  SaturateOnIntegerOverflow=on  InputSameDT=on
  Sum1 : Sum  Inputs=-+|  SaturateOnIntegerOverflow=on  InputSameDT=on
  Sum2 : Sum  Orientation=left  Inputs=|++  SaturateOnIntegerOverflow=on  InputSameDT=on
  Sum3 : Sum  Inputs=-+|  SaturateOnIntegerOverflow=on  InputSameDT=on
  u_demand : Outport  Orientation=left
  wires:
  D/1 -> *D/1, H*D/2
  Sum2/1 -> u_demand/1
  *D/1 -> Sum2/2
  *C/1 -> Sum2/1
  index/1 -> C/1, A/1, D/1, B/1, H/1
  e = refs - y/1 -> *D/2, *B-HD/2
  C/1 -> *C/1, H*C/2
  Estimated state/1 -> *A-HC/2, *C/2
  Sum/1 -> Estimated state/1
  *A-HC/1 -> Sum/3
  *B-HD/1 -> Sum/2
  *H/1 -> Sum/1
  u_measured/1 -> *H/2
  H/1 -> *H/1, H*D/1, H*C/1
  H*D/1 -> Sum1/1
  B/1 -> Sum1/2
  Sum1/1 -> *B-HD/1
  A/1 -> Sum3/2
  Sum3/1 -> *A-HC/1
  H*C/1 -> Sum3/1

== system temp/1D Controller Blend: u=(1-L).K1.y+L.K2.y/K2 ==
  e = refs - y : Inport  Orientation=left
  index : Inport  Port=2
  u_measured : Inport  Orientation=left  Port=3
  *A-HC : Product  Multiplication=Matrix(*)  SaturateOnIntegerOverflow=on  InputSameDT=on
  *B-HD : Product  Orientation=left  Multiplication=Matrix(*)  SaturateOnIntegerOverflow=on  InputSameDT=on
  *C : Product  Orientation=left  Multiplication=Matrix(*)  SaturateOnIntegerOverflow=on  InputSameDT=on
  *D : Product  Orientation=left  Multiplication=Matrix(*)  SaturateOnIntegerOverflow=on  InputSameDT=on
  *H : Product  Orientation=left  Multiplication=Matrix(*)  SaturateOnIntegerOverflow=on  InputSameDT=on
  A : simulink3/Functions & Tables/Direct Look-Up Table (n-D)  maskTabDims=3  explicitNumDims=3  outDims=2-D Matrix  tabIsInput=off  mxTable=A  clipFlag=Warning
  B : simulink3/Functions & Tables/Direct Look-Up Table (n-D)  maskTabDims=3  explicitNumDims=3  outDims=2-D Matrix  tabIsInput=off  mxTable=B  clipFlag=Warning
  C : simulink3/Functions & Tables/Direct Look-Up Table (n-D)  maskTabDims=3  explicitNumDims=3  outDims=2-D Matrix  tabIsInput=off  mxTable=C  clipFlag=Warning
  D : simulink3/Functions & Tables/Direct Look-Up Table (n-D)  maskTabDims=3  explicitNumDims=3  outDims=2-D Matrix  tabIsInput=off  mxTable=D  clipFlag=Warning
  Estimated state : Integrator  Orientation=left  InitialCondition=x_initial
  H : simulink3/Functions & Tables/Direct Look-Up Table (n-D)  maskTabDims=3  explicitNumDims=3  outDims=2-D Matrix  tabIsInput=off  mxTable=H  clipFlag=Warning
  H*C : Product  Multiplication=Matrix(*)  SaturateOnIntegerOverflow=on  InputSameDT=on
  H*D : Product  Multiplication=Matrix(*)  SaturateOnIntegerOverflow=on  InputSameDT=on
  Sum : Sum  Orientation=left  Inputs=+++  SaturateOnIntegerOverflow=on  InputSameDT=on
  Sum1 : Sum  Inputs=-+|  SaturateOnIntegerOverflow=on  InputSameDT=on
  Sum2 : Sum  Orientation=left  Inputs=|++  SaturateOnIntegerOverflow=on  InputSameDT=on
  Sum3 : Sum  Inputs=-+|  SaturateOnIntegerOverflow=on  InputSameDT=on
  u_demand : Outport  Orientation=left
  wires:
  H*C/1 -> Sum3/1
  Sum3/1 -> *A-HC/1
  A/1 -> Sum3/2
  Sum1/1 -> *B-HD/1
  B/1 -> Sum1/2
  H*D/1 -> Sum1/1
  H/1 -> H*C/1, H*D/1, *H/1
  u_measured/1 -> *H/2
  *H/1 -> Sum/1
  *B-HD/1 -> Sum/2
  *A-HC/1 -> Sum/3
  Sum/1 -> Estimated state/1
  Estimated state/1 -> *C/2, *A-HC/2
  C/1 -> H*C/2, *C/1
  e = refs - y/1 -> *B-HD/2, *D/2
  index/1 -> H/1, B/1, D/1, A/1, C/1
  *C/1 -> Sum2/1
  *D/1 -> Sum2/2
  Sum2/1 -> u_demand/1
  D/1 -> H*D/2, *D/1

== system temp/1D Controller Blend: u=(1-L).K1.y+L.K2.y/K3 ==
  e = refs - y : Inport  Orientation=left
  index : Inport  Port=2
  u_measured : Inport  Orientation=left  Port=3
  *A-HC : Product  Multiplication=Matrix(*)  SaturateOnIntegerOverflow=on  InputSameDT=on
  *B-HD : Product  Orientation=left  Multiplication=Matrix(*)  SaturateOnIntegerOverflow=on  InputSameDT=on
  *C : Product  Orientation=left  Multiplication=Matrix(*)  SaturateOnIntegerOverflow=on  InputSameDT=on
  *D : Product  Orientation=left  Multiplication=Matrix(*)  SaturateOnIntegerOverflow=on  InputSameDT=on
  *H : Product  Orientation=left  Multiplication=Matrix(*)  SaturateOnIntegerOverflow=on  InputSameDT=on
  A : simulink/Look-Up Tables/Direct Look-Up Table (n-D)  maskTabDims=3  explicitNumDims=3  outDims=2-D Matrix  tabIsInput=off  mxTable=A  clipFlag=Warning
  B : simulink/Look-Up Tables/Direct Look-Up Table (n-D)  maskTabDims=3  explicitNumDims=3  outDims=2-D Matrix  tabIsInput=off  mxTable=B  clipFlag=Warning
  C : simulink/Look-Up Tables/Direct Look-Up Table (n-D)  maskTabDims=3  explicitNumDims=3  outDims=2-D Matrix  tabIsInput=off  mxTable=C  clipFlag=Warning
  D : simulink/Look-Up Tables/Direct Look-Up Table (n-D)  maskTabDims=3  explicitNumDims=3  outDims=2-D Matrix  tabIsInput=off  mxTable=D  clipFlag=Warning
  Estimated state : Integrator  Orientation=left  InitialCondition=x_initial
  H : simulink/Look-Up Tables/Direct Look-Up Table (n-D)  maskTabDims=3  explicitNumDims=3  outDims=2-D Matrix  tabIsInput=off  mxTable=H  clipFlag=Warning
  H*C : Product  Multiplication=Matrix(*)  SaturateOnIntegerOverflow=on  InputSameDT=on
  H*D : Product  Multiplication=Matrix(*)  SaturateOnIntegerOverflow=on  InputSameDT=on
  Sum : Sum  Orientation=left  Inputs=+++  SaturateOnIntegerOverflow=on  InputSameDT=on
  Sum1 : Sum  Inputs=-+|  SaturateOnIntegerOverflow=on  InputSameDT=on
  Sum2 : Sum  Orientation=left  Inputs=|++  SaturateOnIntegerOverflow=on  InputSameDT=on
  Sum3 : Sum  Inputs=-+|  SaturateOnIntegerOverflow=on  InputSameDT=on
  u_demand : Outport  Orientation=left
  wires:
  D/1 -> *D/1, H*D/2
  Sum2/1 -> u_demand/1
  *D/1 -> Sum2/2
  *C/1 -> Sum2/1
  index/1 -> C/1, A/1, D/1, B/1, H/1
  e = refs - y/1 -> *D/2, *B-HD/2
  C/1 -> *C/1, H*C/2
  Estimated state/1 -> *A-HC/2, *C/2
  Sum/1 -> Estimated state/1
  *A-HC/1 -> Sum/3
  *B-HD/1 -> Sum/2
  *H/1 -> Sum/1
  u_measured/1 -> *H/2
  H/1 -> *H/1, H*D/1, H*C/1
  H*D/1 -> Sum1/1
  B/1 -> Sum1/2
  Sum1/1 -> *B-HD/1
  A/1 -> Sum3/2
  Sum3/1 -> *A-HC/1
  H*C/1 -> Sum3/1

== system temp/1D Observer Form [A(v),B(v),C(v),F(v),H(v)]/[A,B,C,F,H] ==
  y-y_dem : Inport
  AoA : Inport  Port=2  PortDimensions=2
  u_meas : Inport  Port=3
  *A : Product  Multiplication=Matrix(*)  SaturateOnIntegerOverflow=on  InputSameDT=on
  *B : Product  Multiplication=Matrix(*)  SaturateOnIntegerOverflow=on  InputSameDT=on
  *C : Product  Multiplication=Matrix(*)  SaturateOnIntegerOverflow=on  InputSameDT=on
  *F : Product  Orientation=left  Multiplication=Matrix(*)  SaturateOnIntegerOverflow=on  InputSameDT=on
  *H : Product  Orientation=down  Multiplication=Matrix(*)  SaturateOnIntegerOverflow=on  InputSameDT=on
  A : aerolibschedule/Interpolate Matrix(x)  matrix=A
  B : aerolibschedule/Interpolate Matrix(x)  matrix=B
  C : aerolibschedule/Interpolate Matrix(x)  matrix=C
  F : aerolibschedule/Interpolate Matrix(x)  matrix=F
  H : aerolibschedule/Interpolate Matrix(x)  matrix=H
  Sum : Sum  Orientation=left  Inputs=+|+  SaturateOnIntegerOverflow=on  InputSameDT=on
  Sum1 : Sum  Orientation=down  Inputs=++|  SaturateOnIntegerOverflow=on  InputSameDT=on
  Sum2 : Sum  Orientation=down  Inputs=|++  SaturateOnIntegerOverflow=on  InputSameDT=on
  estimated state : Integrator  Orientation=left  InitialCondition=x_initial
  u_dem : Outport
  wires:
  u_meas/1 -> *B/2
  AoA/1 -> A/1, C/1, F/1, B/1, H/1
  y-y_dem/1 -> Sum2/1
  H/1 -> *H/1
  B/1 -> *B/1
  F/1 -> *F/1
  C/1 -> *C/1
  A/1 -> *A/1
  *C/1 -> Sum2/2
  Sum2/1 -> *H/2
  *H/1 -> Sum1/2
  Sum1/1 -> Sum/1
  *B/1 -> Sum1/1
  *F/1 -> u_dem/1
  *A/1 -> Sum/2
  estimated state/1 -> *C/2, *A/2, *F/2
  Sum/1 -> estimated state/1

== system temp/1D Self-Conditioned [A(v),B(v),C(v),D(v)]/Controller ==
  y : Inport  Orientation=left
  idx_v,lam_v : Inport  Port=2  PortDimensions=2
  u_measured : Inport  Orientation=left  Port=3
  *A-HC : Product  Multiplication=Matrix(*)  SaturateOnIntegerOverflow=on  InputSameDT=on
  *B-HD : Product  Orientation=left  Multiplication=Matrix(*)  SaturateOnIntegerOverflow=on  InputSameDT=on
  *C : Product  Orientation=left  Multiplication=Matrix(*)  SaturateOnIntegerOverflow=on  InputSameDT=on
  *D : Product  Orientation=left  Multiplication=Matrix(*)  SaturateOnIntegerOverflow=on  InputSameDT=on
  *H : Product  Orientation=left  Multiplication=Matrix(*)  SaturateOnIntegerOverflow=on  InputSameDT=on
  A : aerolibschedule/Interpolate Matrix(x)  matrix=A
  B : aerolibschedule/Interpolate Matrix(x)  matrix=B
  C : aerolibschedule/Interpolate Matrix(x)  matrix=C
  D : aerolibschedule/Interpolate Matrix(x)  matrix=D
  Estimated state : Integrator  Orientation=left  InitialCondition=x_initial
  H : aerolibschedule/Interpolate Matrix(x)  matrix=H
  H*C : Product  Multiplication=Matrix(*)  SaturateOnIntegerOverflow=on  InputSameDT=on
  H*D : Product  Multiplication=Matrix(*)  SaturateOnIntegerOverflow=on  InputSameDT=on
  Sum : Sum  Orientation=left  Inputs=+++  SaturateOnIntegerOverflow=on  InputSameDT=on
  Sum1 : Sum  Inputs=-+|  SaturateOnIntegerOverflow=on  InputSameDT=on
  Sum2 : Sum  Orientation=left  Inputs=|++  SaturateOnIntegerOverflow=on  InputSameDT=on
  Sum3 : Sum  Inputs=-+|  SaturateOnIntegerOverflow=on  InputSameDT=on
  u_demand : Outport  Orientation=left
  wires:
  D/1 -> *D/1, H*D/2
  Sum2/1 -> u_demand/1
  *D/1 -> Sum2/2
  *C/1 -> Sum2/1
  idx_v,lam_v/1 -> C/1, A/1, D/1, H/1, B/1
  y/1 -> *D/2, *B-HD/2
  C/1 -> *C/1, H*C/2
  Estimated state/1 -> *A-HC/2, *C/2
  Sum/1 -> Estimated state/1
  *A-HC/1 -> Sum/3
  *B-HD/1 -> Sum/2
  *H/1 -> Sum/1
  u_measured/1 -> *H/2
  H/1 -> *H/1, H*D/1, H*C/1
  H*D/1 -> Sum1/1
  B/1 -> Sum1/2
  Sum1/1 -> *B-HD/1
  A/1 -> Sum3/2
  Sum3/1 -> *A-HC/1
  H*C/1 -> Sum3/1

== system temp/2D Controller [A(v),B(v),C(v),D(v)]/[A,B,C,D] ==
  y : Inport  Orientation=left
  AoA : Inport  Port=2  PortDimensions=2
  Mach : Inport  Port=3  PortDimensions=2
  *A : Product  Multiplication=Matrix(*)  SaturateOnIntegerOverflow=on  InputSameDT=on
  *B : Product  Orientation=left  Multiplication=Matrix(*)  SaturateOnIntegerOverflow=on  InputSameDT=on
  *C : Product  Orientation=left  Multiplication=Matrix(*)  SaturateOnIntegerOverflow=on  InputSameDT=on
  *D : Product  Orientation=left  Multiplication=Matrix(*)  SaturateOnIntegerOverflow=on  InputSameDT=on
  A : aerolibschedule/Interpolate Matrix(x,y)  matrix=A
  B : aerolibschedule/Interpolate Matrix(x,y)  matrix=B
  C : aerolibschedule/Interpolate Matrix(x,y)  matrix=C
  D : aerolibschedule/Interpolate Matrix(x,y)  matrix=D
  Estimated state : Integrator  Orientation=left  InitialCondition=x_initial
  Sum : Sum  Orientation=left  Inputs=|++  SaturateOnIntegerOverflow=on  InputSameDT=on
  Sum2 : Sum  Orientation=left  Inputs=|++  SaturateOnIntegerOverflow=on  InputSameDT=on
  u : Outport  Orientation=left
  wires:
  Sum/1 -> Estimated state/1
  Estimated state/1 -> *C/2, *A/2
  *A/1 -> Sum/2
  *B/1 -> Sum/1
  A/1 -> *A/1
  C/1 -> *C/1
  B/1 -> *B/1
  y/1 -> *B/2, *D/2
  AoA/1 -> C/1, A/1, D/1, B/1
  Mach/1 -> C/2, A/2, D/2, B/2
  *C/1 -> Sum2/1
  *D/1 -> Sum2/2
  Sum2/1 -> u/1
  D/1 -> *D/1

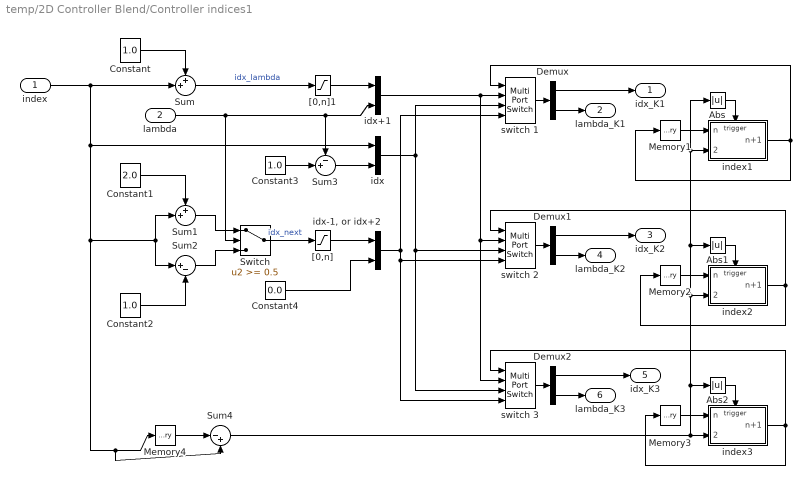
== system temp/2D Controller Blend/Controller indices1 ==
  index : Inport
  lambda : Inport  Port=2
  Abs : Abs  SaturateOnIntegerOverflow=on
  Abs1 : Abs  SaturateOnIntegerOverflow=on
  Abs2 : Abs  SaturateOnIntegerOverflow=on
  Constant : Constant  Value=1.0
  Constant1 : Constant  Value=2.0
  Constant2 : Constant  Value=1.0
  Constant3 : Constant  Value=1.0
  Constant4 : Constant  Value=0.0
  Demux : Demux  Outputs=2
  Demux1 : Demux  Outputs=2
  Demux2 : Demux  Outputs=2
  Memory{1..4} (4 alike) : Memory
  Sum : Sum  Inputs=++|  SaturateOnIntegerOverflow=on  InputSameDT=on
  Sum1 : Sum  Inputs=++|  SaturateOnIntegerOverflow=on  InputSameDT=on
  Sum2 : Sum  Inputs=|+-  SaturateOnIntegerOverflow=on  InputSameDT=on
  Sum3 : Sum  Inputs=-+|  SaturateOnIntegerOverflow=on  InputSameDT=on
  Sum4 : Sum  Inputs=|-+  SaturateOnIntegerOverflow=on  InputSameDT=on
  Switch : Switch  Threshold=0.5  SaturateOnIntegerOverflow=on  InputSameDT=on
  "[0,n]" : Saturate  UpperLimit=length(breakpoints_v1)-1  LowerLimit=0
  "[0,n]1" : Saturate  UpperLimit=length(breakpoints_v1)-1  LowerLimit=0
  idx : Mux  Inputs=2
  idx+1 : Mux  Inputs=2
  "idx-1, or idx+2" : Mux  Inputs=2
  index1 : Subsystem  TreatAsAtomicUnit=on
  index2 : Subsystem  TreatAsAtomicUnit=on
  index3 : Subsystem  TreatAsAtomicUnit=on
  switch 1 : MultiPortSwitch  Inputs=3  SaturateOnIntegerOverflow=on  InputSameDT=on
  switch 2 : MultiPortSwitch  Inputs=3  SaturateOnIntegerOverflow=on  InputSameDT=on
  switch 3 : MultiPortSwitch  Inputs=3  SaturateOnIntegerOverflow=on  InputSameDT=on
  idx_K1 : Outport
  lambda_K1 : Outport  Port=2
  idx_K2 : Outport  Port=3
  lambda_K2 : Outport  Port=4
  idx_K3 : Outport  Port=5
  lambda_K3 : Outport  Port=6
  wires:
  Abs2/1 -> index3/Trigger
  Abs1/1 -> index2/Trigger
  Abs/1 -> index1/Trigger
  Sum4/1 -> Abs2/1, Abs1/1, Abs/1, index1/2(rise/fall), index2/2(rise/fall), index3/2(rise/fall)
  Memory4/1 -> Sum4/1
  "[0,n]1"/1 -> idx+1/1
  "[0,n]"/1 -> "idx-1, or idx+2"/1
  Demux2/2 -> lambda_K3/1
  Demux2/1 -> idx_K3/1
  switch 3/1 -> Demux2/1
  Demux1/2 -> lambda_K2/1
  Demux1/1 -> idx_K2/1
  switch 2/1 -> Demux1/1
  Demux/2 -> lambda_K1/1
  Demux/1 -> idx_K1/1
  switch 1/1 -> Demux/1
  "idx-1, or idx+2"/1 -> switch 3/4, switch 2/4, switch 1/4
  Constant4/1 -> "idx-1, or idx+2"/2
  Switch/1 -> "[0,n]"/1  "idx_next"
  idx/1 -> switch 3/3, switch 2/3, switch 1/3
  Constant3/1 -> Sum3/2
  Sum3/1 -> idx/2
  idx+1/1 -> switch 3/2, switch 2/2, switch 1/2
  lambda/1 -> Switch/2, Sum3/1, idx+1/2
  Sum/1 -> "[0,n]1"/1  "idx_lambda"
  index3/1(n+1) -> Memory3/1, switch 3/1
  index2/1(n+1) -> Memory2/1, switch 2/1
  Memory3/1 -> index3/1(n)
  Memory2/1 -> index2/1(n)
  index1/1(n+1) -> Memory1/1, switch 1/1
  Memory1/1 -> index1/1(n)
  Constant2/1 -> Sum2/2
  Sum2/1 -> Switch/3
  Sum1/1 -> Switch/1
  Constant1/1 -> Sum1/1
  Constant/1 -> Sum/1
  index/1 -> Sum4/2, Memory4/1, Sum2/1, Sum1/2, idx/1, Sum/2
